simulink model "QRD_System"  (R2021a)
settings: Solver=VariableStepAuto  StartTime=0.0  StopTime=800  RelTol=1e-3
undefined symbols (not defined in the file or in its folder): AXI4, Lite
libraries: hdlBasic x268, xbsIndex_r4 x1
(part 2 of 3)

== system QRD_System/Rotation10 ==
  y_in : Inport
  theta_in : Inport  Port=2
  rst : Inport  Port=3
  Q_in : Inport  Port=4
  Constant3 : hdlBasic/Constant  const=0.0  gui_display_data_type=Fixed-point  arith_type=Signed (2's comp)  n_bits=16  bin_pt=13  preci_type=Single  exp_width=8  frac_width=24  explicit_period=off  period=1  XmcBlockStatus=1  maskContainerNames=tabcontainer1  block_type=constant  block_config=sysgen:Constant_config
  Constant4 : hdlBasic/Constant  const=1.0  gui_display_data_type=Boolean  arith_type=Boolean  n_bits=16  bin_pt=14  preci_type=Single  exp_width=8  frac_width=24  explicit_period=off  period=1  XmcBlockStatus=1  maskContainerNames=tabcontainer1  block_type=constant  block_config=sysgen:Constant_config
  Constant5 : hdlBasic/Constant  const=0  gui_display_data_type=Boolean  arith_type=Boolean  n_bits=16  bin_pt=14  preci_type=Single  exp_width=8  frac_width=24  explicit_period=off  period=1  XmcBlockStatus=1  maskContainerNames=tabcontainer1  block_type=constant  block_config=sysgen:Constant_config
  Constant6 : hdlBasic/Constant  const=0  gui_display_data_type=Boolean  arith_type=Boolean  n_bits=16  bin_pt=13  preci_type=Single  exp_width=8  frac_width=24  explicit_period=off  period=1  XmcBlockStatus=1  maskContainerNames=tabcontainer1  block_type=constant  block_config=sysgen:Constant_config
  Constant7 : hdlBasic/Constant  const=0.0  gui_display_data_type=Fixed-point  arith_type=Signed (2's comp)  n_bits=16  bin_pt=0  preci_type=Single  exp_width=8  frac_width=24  explicit_period=off  period=1  XmcBlockStatus=1  maskContainerNames=tabcontainer1  block_type=constant  block_config=sysgen:Constant_config
  Delay1 : hdlBasic/Delay  rst=off  en=off  latency=42  reg_retiming=off  XmcBlockStatus=1  maskContainerNames=group1  block_type=delay  block_config=sysgen:Delay_config
  Delay5 : hdlBasic/Delay  rst=off  en=off  latency=42  reg_retiming=off  XmcBlockStatus=1  maskContainerNames=group1  block_type=delay  block_config=sysgen:Delay_config
  Mux : hdlBasic/Mux  inputs=2  en=off  latency=0  precision=Full  arith_type=Unsigned  n_bits=16  bin_pt=14  quantization=Truncate  overflow=Wrap  XmcBlockStatus=1  maskContainerNames=tabcontainer1  block_type=mux  block_config=sysgen:Mux_config
  Mux2 : hdlBasic/Mux  inputs=2  en=off  latency=0  precision=Full  arith_type=Unsigned  n_bits=16  bin_pt=14  quantization=Truncate  overflow=Wrap  XmcBlockStatus=1  maskContainerNames=tabcontainer1  block_type=mux  block_config=sysgen:Mux_config
  Register : hdlBasic/Register  init=0  rst=on  en=off  XmcBlockStatus=1  maskContainerNames=tabcontainer1  block_type=register  block_config=sysgen:Register_config
  Scope6 : Scope
  Terminator{1..6} (6 alike) : Terminator
  Vitis HLS2 : hdlBasic/Vitis HLS  anytable='C:\ELEC522\hl116\Project5\project5_final\Vitis_HLS\project5_final_hls\solution1'  fast_sim=off  display_datatype=off  rate_propagation_method=Simulink system period  model_file_path=''  latency=1  block_type=vitis_hls
      settings: infoedit=This block allows including C,C++ and SystemC source files in System Generator for DSP designs.
  theta_out : Outport
  y_out : Outport  Port=2
  x_out : Outport  Port=3
  sel_out : Outport  Port=4
  Q_out : Outport  Port=5
  rst_out : Outport  Port=6
  wires:
  Mux/1 -> Mux2/3, Register/1
  Vitis HLS2/4 -> x_out/1, Mux/3
  y_in/1 -> Vitis HLS2/5
  Constant3/1 -> Mux/2
  Vitis HLS2/5 -> sel_out/1, Mux/1
  Vitis HLS2/6 -> y_out/1
  rst/1 -> Delay1/1, Register/2, Mux2/1
  Register/1 -> Vitis HLS2/4
  Constant6/1 -> Vitis HLS2/3
  Constant7/1 -> Vitis HLS2/7
  Constant4/1 -> Vitis HLS2/2
  Constant5/1 -> Vitis HLS2/1
  Vitis HLS2/1 -> Terminator3/1
  Vitis HLS2/2 -> Terminator1/1
  Vitis HLS2/3 -> Terminator6/1
  Vitis HLS2/7 -> Terminator2/1
  Vitis HLS2/8 -> Terminator5/1
  Vitis HLS2/9 -> Terminator4/1
  Mux2/1 -> Q_out/1, Scope6/1
  Q_in/1 -> Mux2/2
  Delay5/1 -> Vitis HLS2/6, theta_out/1
  theta_in/1 -> Delay5/1
  Delay1/1 -> rst_out/1

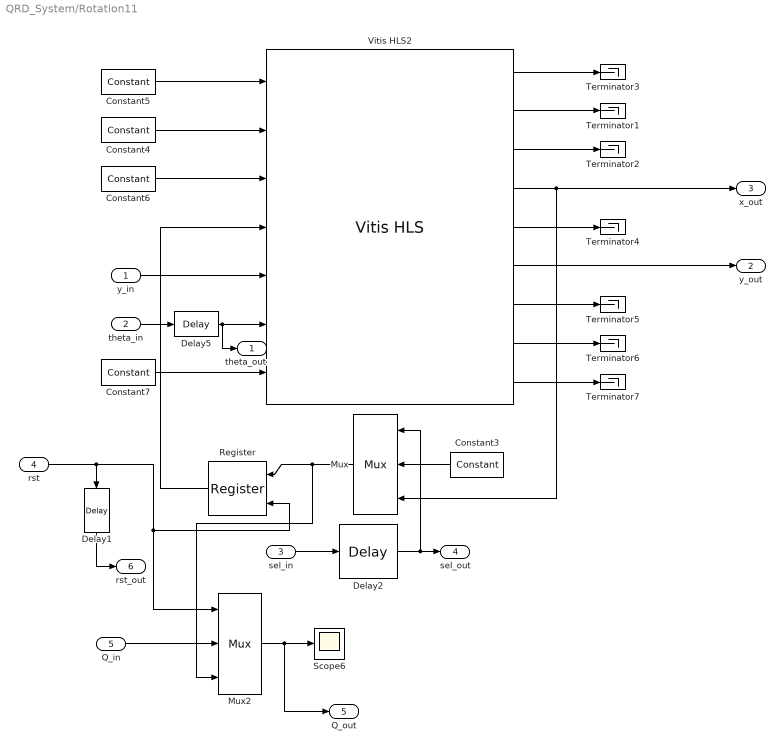
== system QRD_System/Rotation11 ==
  y_in : Inport
  theta_in : Inport  Port=2
  sel_in : Inport  Port=3
  rst : Inport  Port=4
  Q_in : Inport  Port=5
  Constant3 : hdlBasic/Constant  const=0.0  gui_display_data_type=Fixed-point  arith_type=Signed (2's comp)  n_bits=16  bin_pt=13  preci_type=Single  exp_width=8  frac_width=24  explicit_period=off  period=1  XmcBlockStatus=1  maskContainerNames=tabcontainer1  block_type=constant  block_config=sysgen:Constant_config
  Constant4 : hdlBasic/Constant  const=1.0  gui_display_data_type=Boolean  arith_type=Boolean  n_bits=16  bin_pt=14  preci_type=Single  exp_width=8  frac_width=24  explicit_period=off  period=1  XmcBlockStatus=1  maskContainerNames=tabcontainer1  block_type=constant  block_config=sysgen:Constant_config
  Constant5 : hdlBasic/Constant  const=0  gui_display_data_type=Boolean  arith_type=Boolean  n_bits=16  bin_pt=14  preci_type=Single  exp_width=8  frac_width=24  explicit_period=off  period=1  XmcBlockStatus=1  maskContainerNames=tabcontainer1  block_type=constant  block_config=sysgen:Constant_config
  Constant6 : hdlBasic/Constant  const=0  gui_display_data_type=Boolean  arith_type=Boolean  n_bits=16  bin_pt=13  preci_type=Single  exp_width=8  frac_width=24  explicit_period=off  period=1  XmcBlockStatus=1  maskContainerNames=tabcontainer1  block_type=constant  block_config=sysgen:Constant_config
  Constant7 : hdlBasic/Constant  const=0.0  gui_display_data_type=Fixed-point  arith_type=Signed (2's comp)  n_bits=16  bin_pt=0  preci_type=Single  exp_width=8  frac_width=24  explicit_period=off  period=1  XmcBlockStatus=1  maskContainerNames=tabcontainer1  block_type=constant  block_config=sysgen:Constant_config
  Delay1 : hdlBasic/Delay  rst=off  en=off  latency=42  reg_retiming=off  XmcBlockStatus=1  maskContainerNames=group1  block_type=delay  block_config=sysgen:Delay_config
  Delay2 : hdlBasic/Delay  rst=off  en=off  latency=43  reg_retiming=off  XmcBlockStatus=1  maskContainerNames=group1  block_type=delay  block_config=sysgen:Delay_config
  Delay5 : hdlBasic/Delay  rst=off  en=off  latency=42  reg_retiming=off  XmcBlockStatus=1  maskContainerNames=group1  block_type=delay  block_config=sysgen:Delay_config
  Mux : hdlBasic/Mux  inputs=2  en=off  latency=0  precision=Full  arith_type=Unsigned  n_bits=16  bin_pt=14  quantization=Truncate  overflow=Wrap  XmcBlockStatus=1  maskContainerNames=tabcontainer1  block_type=mux  block_config=sysgen:Mux_config
  Mux2 : hdlBasic/Mux  inputs=2  en=off  latency=0  precision=Full  arith_type=Unsigned  n_bits=16  bin_pt=14  quantization=Truncate  overflow=Wrap  XmcBlockStatus=1  maskContainerNames=tabcontainer1  block_type=mux  block_config=sysgen:Mux_config
  Register : hdlBasic/Register  init=0  rst=on  en=off  XmcBlockStatus=1  maskContainerNames=tabcontainer1  block_type=register  block_config=sysgen:Register_config
  Scope6 : Scope
  Terminator{1..7} (7 alike) : Terminator
  Vitis HLS2 : hdlBasic/Vitis HLS  anytable='C:\ELEC522\hl116\Project5\project5_final\Vitis_HLS\project5_final_hls\solution1'  fast_sim=off  display_datatype=off  rate_propagation_method=Simulink system period  model_file_path=''  latency=1  block_type=vitis_hls
      settings: infoedit=This block allows including C,C++ and SystemC source files in System Generator for DSP designs.
  theta_out : Outport
  y_out : Outport  Port=2
  x_out : Outport  Port=3
  sel_out : Outport  Port=4
  Q_out : Outport  Port=5
  rst_out : Outport  Port=6
  wires:
  Mux/1 -> Mux2/3, Register/1
  Vitis HLS2/4 -> x_out/1, Mux/3
  y_in/1 -> Vitis HLS2/5
  Constant3/1 -> Mux/2
  Vitis HLS2/6 -> y_out/1
  theta_in/1 -> Delay5/1
  sel_in/1 -> Delay2/1
  Register/1 -> Vitis HLS2/4
  rst/1 -> Delay1/1, Mux2/1, Register/2
  Delay2/1 -> Mux/1, sel_out/1
  Constant6/1 -> Vitis HLS2/3
  Constant7/1 -> Vitis HLS2/7
  Constant4/1 -> Vitis HLS2/2
  Constant5/1 -> Vitis HLS2/1
  Vitis HLS2/9 -> Terminator7/1
  Vitis HLS2/8 -> Terminator6/1
  Vitis HLS2/7 -> Terminator5/1
  Vitis HLS2/2 -> Terminator1/1
  Vitis HLS2/1 -> Terminator3/1
  Vitis HLS2/3 -> Terminator2/1
  Vitis HLS2/5 -> Terminator4/1
  Mux2/1 -> Q_out/1, Scope6/1
  Q_in/1 -> Mux2/2
  Delay5/1 -> Vitis HLS2/6, theta_out/1
  Delay1/1 -> rst_out/1

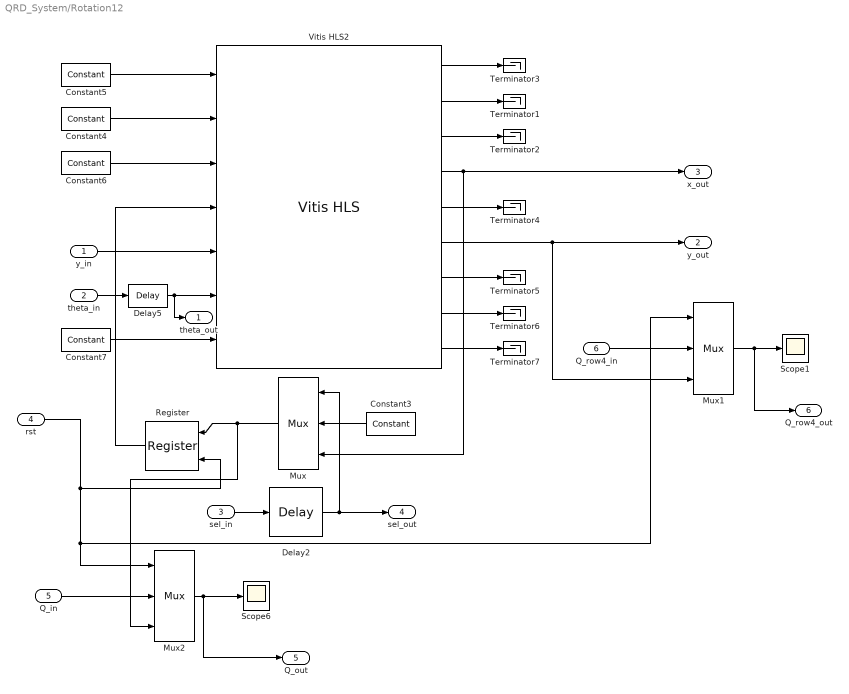
== system QRD_System/Rotation12 ==
  y_in : Inport
  theta_in : Inport  Port=2
  sel_in : Inport  Port=3
  rst : Inport  Port=4
  Q_in : Inport  Port=5
  Q_row4_in : Inport  Port=6
  Constant3 : hdlBasic/Constant  const=0.0  gui_display_data_type=Fixed-point  arith_type=Signed (2's comp)  n_bits=16  bin_pt=13  preci_type=Single  exp_width=8  frac_width=24  explicit_period=off  period=1  XmcBlockStatus=1  maskContainerNames=tabcontainer1  block_type=constant  block_config=sysgen:Constant_config
  Constant4 : hdlBasic/Constant  const=1.0  gui_display_data_type=Boolean  arith_type=Boolean  n_bits=16  bin_pt=14  preci_type=Single  exp_width=8  frac_width=24  explicit_period=off  period=1  XmcBlockStatus=1  maskContainerNames=tabcontainer1  block_type=constant  block_config=sysgen:Constant_config
  Constant5 : hdlBasic/Constant  const=0  gui_display_data_type=Boolean  arith_type=Boolean  n_bits=16  bin_pt=14  preci_type=Single  exp_width=8  frac_width=24  explicit_period=off  period=1  XmcBlockStatus=1  maskContainerNames=tabcontainer1  block_type=constant  block_config=sysgen:Constant_config
  Constant6 : hdlBasic/Constant  const=0  gui_display_data_type=Boolean  arith_type=Boolean  n_bits=16  bin_pt=13  preci_type=Single  exp_width=8  frac_width=24  explicit_period=off  period=1  XmcBlockStatus=1  maskContainerNames=tabcontainer1  block_type=constant  block_config=sysgen:Constant_config
  Constant7 : hdlBasic/Constant  const=0.0  gui_display_data_type=Fixed-point  arith_type=Signed (2's comp)  n_bits=16  bin_pt=0  preci_type=Single  exp_width=8  frac_width=24  explicit_period=off  period=1  XmcBlockStatus=1  maskContainerNames=tabcontainer1  block_type=constant  block_config=sysgen:Constant_config
  Delay2 : hdlBasic/Delay  rst=off  en=off  latency=43  reg_retiming=off  XmcBlockStatus=1  maskContainerNames=group1  block_type=delay  block_config=sysgen:Delay_config
  Delay5 : hdlBasic/Delay  rst=off  en=off  latency=42  reg_retiming=off  XmcBlockStatus=1  maskContainerNames=group1  block_type=delay  block_config=sysgen:Delay_config
  Mux : hdlBasic/Mux  inputs=2  en=off  latency=0  precision=Full  arith_type=Unsigned  n_bits=16  bin_pt=14  quantization=Truncate  overflow=Wrap  XmcBlockStatus=1  maskContainerNames=tabcontainer1  block_type=mux  block_config=sysgen:Mux_config
  Mux1 : hdlBasic/Mux  inputs=2  en=off  latency=0  precision=Full  arith_type=Unsigned  n_bits=16  bin_pt=14  quantization=Truncate  overflow=Wrap  XmcBlockStatus=1  maskContainerNames=tabcontainer1  block_type=mux  block_config=sysgen:Mux_config
  Mux2 : hdlBasic/Mux  inputs=2  en=off  latency=0  precision=Full  arith_type=Unsigned  n_bits=16  bin_pt=14  quantization=Truncate  overflow=Wrap  XmcBlockStatus=1  maskContainerNames=tabcontainer1  block_type=mux  block_config=sysgen:Mux_config
  Register : hdlBasic/Register  init=0  rst=on  en=off  XmcBlockStatus=1  maskContainerNames=tabcontainer1  block_type=register  block_config=sysgen:Register_config
  Scope1 : Scope
  Scope6 : Scope
  Terminator{1..7} (7 alike) : Terminator
  Vitis HLS2 : hdlBasic/Vitis HLS  anytable='C:\ELEC522\hl116\Project5\project5_final\Vitis_HLS\project5_final_hls\solution1'  fast_sim=off  display_datatype=off  rate_propagation_method=Simulink system period  model_file_path=''  latency=1  block_type=vitis_hls
      settings: infoedit=This block allows including C,C++ and SystemC source files in System Generator for DSP designs.
  theta_out : Outport
  y_out : Outport  Port=2
  x_out : Outport  Port=3
  sel_out : Outport  Port=4
  Q_out : Outport  Port=5
  Q_row4_out : Outport  Port=6
  wires:
  Mux/1 -> Mux2/3, Register/1
  Vitis HLS2/4 -> x_out/1, Mux/3
  y_in/1 -> Vitis HLS2/5
  Constant3/1 -> Mux/2
  theta_in/1 -> Delay5/1
  sel_in/1 -> Delay2/1
  Register/1 -> Vitis HLS2/4
  rst/1 -> Mux2/1, Mux1/1, Register/2
  Delay2/1 -> Mux/1, sel_out/1
  Constant6/1 -> Vitis HLS2/3
  Constant7/1 -> Vitis HLS2/7
  Constant4/1 -> Vitis HLS2/2
  Constant5/1 -> Vitis HLS2/1
  Vitis HLS2/3 -> Terminator2/1
  Vitis HLS2/2 -> Terminator1/1
  Vitis HLS2/1 -> Terminator3/1
  Vitis HLS2/5 -> Terminator4/1
  Vitis HLS2/7 -> Terminator5/1
  Vitis HLS2/8 -> Terminator6/1
  Vitis HLS2/9 -> Terminator7/1
  Mux1/1 -> Q_row4_out/1, Scope1/1
  Q_row4_in/1 -> Mux1/2
  Vitis HLS2/6 -> Mux1/3, y_out/1
  Q_in/1 -> Mux2/2
  Mux2/1 -> Q_out/1, Scope6/1
  Delay5/1 -> Vitis HLS2/6, theta_out/1

== system QRD_System/Rotation13 ==
  y_in : Inport
  theta_in : Inport  Port=2
  rst : Inport  Port=3
  Q_in : Inport  Port=4
  Constant3 : hdlBasic/Constant  const=0.0  gui_display_data_type=Fixed-point  arith_type=Signed (2's comp)  n_bits=16  bin_pt=13  preci_type=Single  exp_width=8  frac_width=24  explicit_period=off  period=1  XmcBlockStatus=1  maskContainerNames=tabcontainer1  block_type=constant  block_config=sysgen:Constant_config
  Constant4 : hdlBasic/Constant  const=1.0  gui_display_data_type=Boolean  arith_type=Boolean  n_bits=16  bin_pt=14  preci_type=Single  exp_width=8  frac_width=24  explicit_period=off  period=1  XmcBlockStatus=1  maskContainerNames=tabcontainer1  block_type=constant  block_config=sysgen:Constant_config
  Constant5 : hdlBasic/Constant  const=0  gui_display_data_type=Boolean  arith_type=Boolean  n_bits=16  bin_pt=14  preci_type=Single  exp_width=8  frac_width=24  explicit_period=off  period=1  XmcBlockStatus=1  maskContainerNames=tabcontainer1  block_type=constant  block_config=sysgen:Constant_config
  Constant6 : hdlBasic/Constant  const=0  gui_display_data_type=Boolean  arith_type=Boolean  n_bits=16  bin_pt=13  preci_type=Single  exp_width=8  frac_width=24  explicit_period=off  period=1  XmcBlockStatus=1  maskContainerNames=tabcontainer1  block_type=constant  block_config=sysgen:Constant_config
  Constant7 : hdlBasic/Constant  const=0.0  gui_display_data_type=Fixed-point  arith_type=Signed (2's comp)  n_bits=16  bin_pt=0  preci_type=Single  exp_width=8  frac_width=24  explicit_period=off  period=1  XmcBlockStatus=1  maskContainerNames=tabcontainer1  block_type=constant  block_config=sysgen:Constant_config
  Delay1 : hdlBasic/Delay  rst=off  en=off  latency=42  reg_retiming=off  XmcBlockStatus=1  maskContainerNames=group1  block_type=delay  block_config=sysgen:Delay_config
  Delay5 : hdlBasic/Delay  rst=off  en=off  latency=42  reg_retiming=off  XmcBlockStatus=1  maskContainerNames=group1  block_type=delay  block_config=sysgen:Delay_config
  Mux : hdlBasic/Mux  inputs=2  en=off  latency=0  precision=Full  arith_type=Unsigned  n_bits=16  bin_pt=14  quantization=Truncate  overflow=Wrap  XmcBlockStatus=1  maskContainerNames=tabcontainer1  block_type=mux  block_config=sysgen:Mux_config
  Mux2 : hdlBasic/Mux  inputs=2  en=off  latency=0  precision=Full  arith_type=Unsigned  n_bits=16  bin_pt=14  quantization=Truncate  overflow=Wrap  XmcBlockStatus=1  maskContainerNames=tabcontainer1  block_type=mux  block_config=sysgen:Mux_config
  Register : hdlBasic/Register  init=0  rst=on  en=off  XmcBlockStatus=1  maskContainerNames=tabcontainer1  block_type=register  block_config=sysgen:Register_config
  Scope6 : Scope
  Terminator{1..6} (6 alike) : Terminator
  Vitis HLS2 : hdlBasic/Vitis HLS  anytable='C:\ELEC522\hl116\Project5\project5_final\Vitis_HLS\project5_final_hls\solution1'  fast_sim=off  display_datatype=off  rate_propagation_method=Simulink system period  model_file_path=''  latency=1  block_type=vitis_hls
      settings: infoedit=This block allows including C,C++ and SystemC source files in System Generator for DSP designs.
  theta_out : Outport
  y_out : Outport  Port=2
  x_out : Outport  Port=3
  sel_out : Outport  Port=4
  Q_out : Outport  Port=5
  rst_out : Outport  Port=6
  wires:
  Mux/1 -> Mux2/3, Register/1
  Vitis HLS2/4 -> Mux/3, x_out/1
  y_in/1 -> Vitis HLS2/5
  Constant3/1 -> Mux/2
  Vitis HLS2/5 -> sel_out/1, Mux/1
  Vitis HLS2/6 -> y_out/1
  rst/1 -> Delay1/1, Register/2, Mux2/1
  Register/1 -> Vitis HLS2/4
  Constant6/1 -> Vitis HLS2/3
  Constant7/1 -> Vitis HLS2/7
  Constant4/1 -> Vitis HLS2/2
  Constant5/1 -> Vitis HLS2/1
  Vitis HLS2/7 -> Terminator2/1
  Vitis HLS2/8 -> Terminator5/1
  Vitis HLS2/9 -> Terminator4/1
  Vitis HLS2/3 -> Terminator6/1
  Vitis HLS2/2 -> Terminator1/1
  Vitis HLS2/1 -> Terminator3/1
  Mux2/1 -> Q_out/1, Scope6/1
  Q_in/1 -> Mux2/2
  Delay5/1 -> Vitis HLS2/6, theta_out/1
  theta_in/1 -> Delay5/1
  Delay1/1 -> rst_out/1

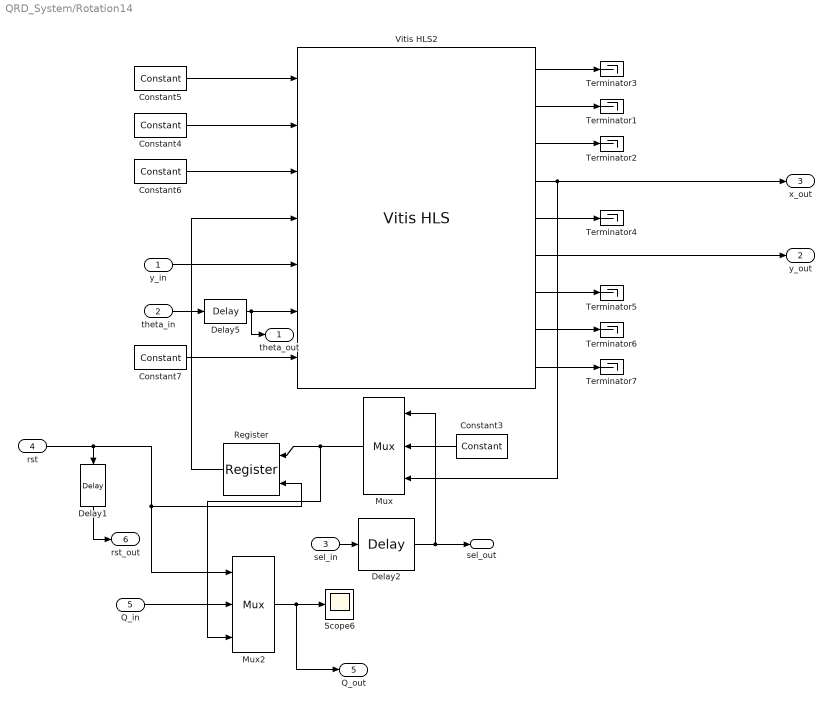
== system QRD_System/Rotation14 ==
  y_in : Inport
  theta_in : Inport  Port=2
  sel_in : Inport  Port=3
  rst : Inport  Port=4
  Q_in : Inport  Port=5
  Constant3 : hdlBasic/Constant  const=0.0  gui_display_data_type=Fixed-point  arith_type=Signed (2's comp)  n_bits=16  bin_pt=13  preci_type=Single  exp_width=8  frac_width=24  explicit_period=off  period=1  XmcBlockStatus=1  maskContainerNames=tabcontainer1  block_type=constant  block_config=sysgen:Constant_config
  Constant4 : hdlBasic/Constant  const=1.0  gui_display_data_type=Boolean  arith_type=Boolean  n_bits=16  bin_pt=14  preci_type=Single  exp_width=8  frac_width=24  explicit_period=off  period=1  XmcBlockStatus=1  maskContainerNames=tabcontainer1  block_type=constant  block_config=sysgen:Constant_config
  Constant5 : hdlBasic/Constant  const=0  gui_display_data_type=Boolean  arith_type=Boolean  n_bits=16  bin_pt=14  preci_type=Single  exp_width=8  frac_width=24  explicit_period=off  period=1  XmcBlockStatus=1  maskContainerNames=tabcontainer1  block_type=constant  block_config=sysgen:Constant_config
  Constant6 : hdlBasic/Constant  const=0  gui_display_data_type=Boolean  arith_type=Boolean  n_bits=16  bin_pt=13  preci_type=Single  exp_width=8  frac_width=24  explicit_period=off  period=1  XmcBlockStatus=1  maskContainerNames=tabcontainer1  block_type=constant  block_config=sysgen:Constant_config
  Constant7 : hdlBasic/Constant  const=0.0  gui_display_data_type=Fixed-point  arith_type=Signed (2's comp)  n_bits=16  bin_pt=0  preci_type=Single  exp_width=8  frac_width=24  explicit_period=off  period=1  XmcBlockStatus=1  maskContainerNames=tabcontainer1  block_type=constant  block_config=sysgen:Constant_config
  Delay1 : hdlBasic/Delay  rst=off  en=off  latency=42  reg_retiming=off  XmcBlockStatus=1  maskContainerNames=group1  block_type=delay  block_config=sysgen:Delay_config
  Delay2 : hdlBasic/Delay  rst=off  en=off  latency=43  reg_retiming=off  XmcBlockStatus=1  maskContainerNames=group1  block_type=delay  block_config=sysgen:Delay_config
  Delay5 : hdlBasic/Delay  rst=off  en=off  latency=42  reg_retiming=off  XmcBlockStatus=1  maskContainerNames=group1  block_type=delay  block_config=sysgen:Delay_config
  Mux : hdlBasic/Mux  inputs=2  en=off  latency=0  precision=Full  arith_type=Unsigned  n_bits=16  bin_pt=14  quantization=Truncate  overflow=Wrap  XmcBlockStatus=1  maskContainerNames=tabcontainer1  block_type=mux  block_config=sysgen:Mux_config
  Mux2 : hdlBasic/Mux  inputs=2  en=off  latency=0  precision=Full  arith_type=Unsigned  n_bits=16  bin_pt=14  quantization=Truncate  overflow=Wrap  XmcBlockStatus=1  maskContainerNames=tabcontainer1  block_type=mux  block_config=sysgen:Mux_config
  Register : hdlBasic/Register  init=0  rst=on  en=off  XmcBlockStatus=1  maskContainerNames=tabcontainer1  block_type=register  block_config=sysgen:Register_config
  Scope6 : Scope
  Terminator{1..7} (7 alike) : Terminator
  Vitis HLS2 : hdlBasic/Vitis HLS  anytable='C:\ELEC522\hl116\Project5\project5_final\Vitis_HLS\project5_final_hls\solution1'  fast_sim=off  display_datatype=off  rate_propagation_method=Simulink system period  model_file_path=''  latency=1  block_type=vitis_hls
      settings: infoedit=This block allows including C,C++ and SystemC source files in System Generator for DSP designs.
  theta_out : Outport
  y_out : Outport  Port=2
  x_out : Outport  Port=3
  sel_out : Outport  Port=4
  Q_out : Outport  Port=5
  rst_out : Outport  Port=6
  wires:
  Mux/1 -> Mux2/3, Register/1
  Vitis HLS2/4 -> Mux/3, x_out/1
  Constant3/1 -> Mux/2
  Vitis HLS2/6 -> y_out/1
  theta_in/1 -> Delay5/1
  Register/1 -> Vitis HLS2/4
  rst/1 -> Delay1/1, Mux2/1, Register/2
  Constant6/1 -> Vitis HLS2/3
  Constant7/1 -> Vitis HLS2/7
  Constant4/1 -> Vitis HLS2/2
  Constant5/1 -> Vitis HLS2/1
  y_in/1 -> Vitis HLS2/5
  Vitis HLS2/7 -> Terminator5/1
  Vitis HLS2/8 -> Terminator6/1
  Vitis HLS2/1 -> Terminator3/1
  Vitis HLS2/2 -> Terminator1/1
  Vitis HLS2/3 -> Terminator2/1
  Vitis HLS2/5 -> Terminator4/1
  Vitis HLS2/9 -> Terminator7/1
  sel_in/1 -> Delay2/1
  Delay2/1 -> sel_out/1, Mux/1
  Mux2/1 -> Q_out/1, Scope6/1
  Q_in/1 -> Mux2/2
  Delay5/1 -> theta_out/1, Vitis HLS2/6
  Delay1/1 -> rst_out/1

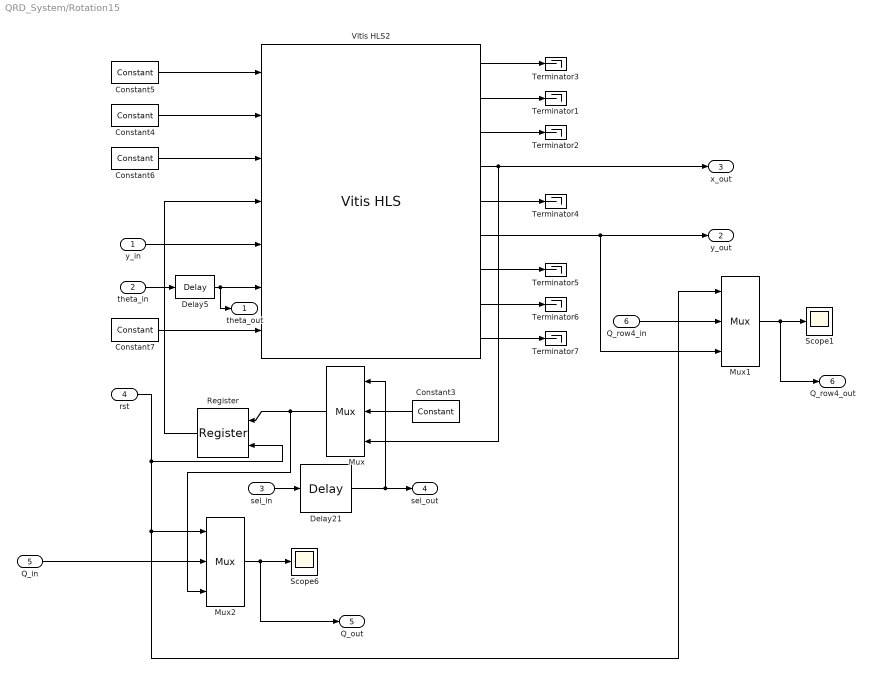
== system QRD_System/Rotation15 ==
  y_in : Inport
  theta_in : Inport  Port=2
  sel_in : Inport  Port=3
  rst : Inport  Port=4
  Q_in : Inport  Port=5
  Q_row4_in : Inport  Port=6
  Constant3 : hdlBasic/Constant  const=0.0  gui_display_data_type=Fixed-point  arith_type=Signed (2's comp)  n_bits=16  bin_pt=13  preci_type=Single  exp_width=8  frac_width=24  explicit_period=off  period=1  XmcBlockStatus=1  maskContainerNames=tabcontainer1  block_type=constant  block_config=sysgen:Constant_config
  Constant4 : hdlBasic/Constant  const=1.0  gui_display_data_type=Boolean  arith_type=Boolean  n_bits=16  bin_pt=14  preci_type=Single  exp_width=8  frac_width=24  explicit_period=off  period=1  XmcBlockStatus=1  maskContainerNames=tabcontainer1  block_type=constant  block_config=sysgen:Constant_config
  Constant5 : hdlBasic/Constant  const=0  gui_display_data_type=Boolean  arith_type=Boolean  n_bits=16  bin_pt=14  preci_type=Single  exp_width=8  frac_width=24  explicit_period=off  period=1  XmcBlockStatus=1  maskContainerNames=tabcontainer1  block_type=constant  block_config=sysgen:Constant_config
  Constant6 : hdlBasic/Constant  const=0  gui_display_data_type=Boolean  arith_type=Boolean  n_bits=16  bin_pt=13  preci_type=Single  exp_width=8  frac_width=24  explicit_period=off  period=1  XmcBlockStatus=1  maskContainerNames=tabcontainer1  block_type=constant  block_config=sysgen:Constant_config
  Constant7 : hdlBasic/Constant  const=0.0  gui_display_data_type=Fixed-point  arith_type=Signed (2's comp)  n_bits=16  bin_pt=0  preci_type=Single  exp_width=8  frac_width=24  explicit_period=off  period=1  XmcBlockStatus=1  maskContainerNames=tabcontainer1  block_type=constant  block_config=sysgen:Constant_config
  Delay21 : hdlBasic/Delay  rst=off  en=off  latency=43  reg_retiming=off  XmcBlockStatus=1  maskContainerNames=group1  block_type=delay  block_config=sysgen:Delay_config
  Delay5 : hdlBasic/Delay  rst=off  en=off  latency=42  reg_retiming=off  XmcBlockStatus=1  maskContainerNames=group1  block_type=delay  block_config=sysgen:Delay_config
  Mux : hdlBasic/Mux  inputs=2  en=off  latency=0  precision=Full  arith_type=Unsigned  n_bits=16  bin_pt=14  quantization=Truncate  overflow=Wrap  XmcBlockStatus=1  maskContainerNames=tabcontainer1  block_type=mux  block_config=sysgen:Mux_config
  Mux1 : hdlBasic/Mux  inputs=2  en=off  latency=0  precision=Full  arith_type=Unsigned  n_bits=16  bin_pt=14  quantization=Truncate  overflow=Wrap  XmcBlockStatus=1  maskContainerNames=tabcontainer1  block_type=mux  block_config=sysgen:Mux_config
  Mux2 : hdlBasic/Mux  inputs=2  en=off  latency=0  precision=Full  arith_type=Unsigned  n_bits=16  bin_pt=14  quantization=Truncate  overflow=Wrap  XmcBlockStatus=1  maskContainerNames=tabcontainer1  block_type=mux  block_config=sysgen:Mux_config
  Register : hdlBasic/Register  init=0  rst=on  en=off  XmcBlockStatus=1  maskContainerNames=tabcontainer1  block_type=register  block_config=sysgen:Register_config
  Scope1 : Scope
  Scope6 : Scope
  Terminator{1..7} (7 alike) : Terminator
  Vitis HLS2 : hdlBasic/Vitis HLS  anytable='C:\ELEC522\hl116\Project5\project5_final\Vitis_HLS\project5_final_hls\solution1'  fast_sim=off  display_datatype=off  rate_propagation_method=Simulink system period  model_file_path=''  latency=1  block_type=vitis_hls
      settings: infoedit=This block allows including C,C++ and SystemC source files in System Generator for DSP designs.
  theta_out : Outport
  y_out : Outport  Port=2
  x_out : Outport  Port=3
  sel_out : Outport  Port=4
  Q_out : Outport  Port=5
  Q_row4_out : Outport  Port=6
  wires:
  Mux/1 -> Mux2/3, Register/1
  Vitis HLS2/4 -> x_out/1, Mux/3
  y_in/1 -> Vitis HLS2/5
  Constant3/1 -> Mux/2
  theta_in/1 -> Delay5/1
  sel_in/1 -> Delay21/1
  Register/1 -> Vitis HLS2/4
  Delay21/1 -> Mux/1, sel_out/1
  Constant6/1 -> Vitis HLS2/3
  Constant7/1 -> Vitis HLS2/7
  Constant4/1 -> Vitis HLS2/2
  Constant5/1 -> Vitis HLS2/1
  Vitis HLS2/1 -> Terminator3/1
  Vitis HLS2/2 -> Terminator1/1
  Vitis HLS2/3 -> Terminator2/1
  Vitis HLS2/5 -> Terminator4/1
  Vitis HLS2/7 -> Terminator5/1
  Vitis HLS2/8 -> Terminator6/1
  Vitis HLS2/9 -> Terminator7/1
  Q_in/1 -> Mux2/2
  rst/1 -> Mux1/1, Mux2/1, Register/2
  Mux1/1 -> Q_row4_out/1, Scope1/1
  Q_row4_in/1 -> Mux1/2
  Vitis HLS2/6 -> Mux1/3, y_out/1
  Mux2/1 -> Q_out/1, Scope6/1
  Delay5/1 -> theta_out/1, Vitis HLS2/6

== system QRD_System/Rotation16 ==
  y_in : Inport
  theta_in : Inport  Port=2
  rst : Inport  Port=3
  Q_in : Inport  Port=4
  Constant3 : hdlBasic/Constant  const=0.0  gui_display_data_type=Fixed-point  arith_type=Signed (2's comp)  n_bits=16  bin_pt=13  preci_type=Single  exp_width=8  frac_width=24  explicit_period=off  period=1  XmcBlockStatus=1  maskContainerNames=tabcontainer1  block_type=constant  block_config=sysgen:Constant_config
  Constant4 : hdlBasic/Constant  const=1.0  gui_display_data_type=Boolean  arith_type=Boolean  n_bits=16  bin_pt=14  preci_type=Single  exp_width=8  frac_width=24  explicit_period=off  period=1  XmcBlockStatus=1  maskContainerNames=tabcontainer1  block_type=constant  block_config=sysgen:Constant_config
  Constant5 : hdlBasic/Constant  const=0  gui_display_data_type=Boolean  arith_type=Boolean  n_bits=16  bin_pt=14  preci_type=Single  exp_width=8  frac_width=24  explicit_period=off  period=1  XmcBlockStatus=1  maskContainerNames=tabcontainer1  block_type=constant  block_config=sysgen:Constant_config
  Constant6 : hdlBasic/Constant  const=0  gui_display_data_type=Boolean  arith_type=Boolean  n_bits=16  bin_pt=13  preci_type=Single  exp_width=8  frac_width=24  explicit_period=off  period=1  XmcBlockStatus=1  maskContainerNames=tabcontainer1  block_type=constant  block_config=sysgen:Constant_config
  Constant7 : hdlBasic/Constant  const=0.0  gui_display_data_type=Fixed-point  arith_type=Signed (2's comp)  n_bits=16  bin_pt=0  preci_type=Single  exp_width=8  frac_width=24  explicit_period=off  period=1  XmcBlockStatus=1  maskContainerNames=tabcontainer1  block_type=constant  block_config=sysgen:Constant_config
  Delay1 : hdlBasic/Delay  rst=off  en=off  latency=42  reg_retiming=off  XmcBlockStatus=1  maskContainerNames=group1  block_type=delay  block_config=sysgen:Delay_config
  Delay5 : hdlBasic/Delay  rst=off  en=off  latency=42  reg_retiming=off  XmcBlockStatus=1  maskContainerNames=group1  block_type=delay  block_config=sysgen:Delay_config
  Mux : hdlBasic/Mux  inputs=2  en=off  latency=0  precision=Full  arith_type=Unsigned  n_bits=16  bin_pt=14  quantization=Truncate  overflow=Wrap  XmcBlockStatus=1  maskContainerNames=tabcontainer1  block_type=mux  block_config=sysgen:Mux_config
  Mux2 : hdlBasic/Mux  inputs=2  en=off  latency=0  precision=Full  arith_type=Unsigned  n_bits=16  bin_pt=14  quantization=Truncate  overflow=Wrap  XmcBlockStatus=1  maskContainerNames=tabcontainer1  block_type=mux  block_config=sysgen:Mux_config
  Register : hdlBasic/Register  init=0  rst=on  en=off  XmcBlockStatus=1  maskContainerNames=tabcontainer1  block_type=register  block_config=sysgen:Register_config
  Scope6 : Scope
  Terminator{1..6} (6 alike) : Terminator
  Vitis HLS2 : hdlBasic/Vitis HLS  anytable='C:\ELEC522\hl116\Project5\project5_final\Vitis_HLS\project5_final_hls\solution1'  fast_sim=off  display_datatype=off  rate_propagation_method=Simulink system period  model_file_path=''  latency=1  block_type=vitis_hls
      settings: infoedit=This block allows including C,C++ and SystemC source files in System Generator for DSP designs.
  theta_out : Outport
  y_out : Outport  Port=2
  x_out : Outport  Port=3
  sel_out : Outport  Port=4
  Q_out : Outport  Port=5
  rst_out : Outport  Port=6
  wires:
  Mux/1 -> Mux2/3, Register/1
  Vitis HLS2/4 -> Mux/3, x_out/1
  y_in/1 -> Vitis HLS2/5
  Constant3/1 -> Mux/2
  Vitis HLS2/5 -> Mux/1, sel_out/1
  Vitis HLS2/6 -> y_out/1
  rst/1 -> Delay1/1, Register/2, Mux2/1
  Register/1 -> Vitis HLS2/4
  Constant6/1 -> Vitis HLS2/3
  Constant7/1 -> Vitis HLS2/7
  Constant4/1 -> Vitis HLS2/2
  Constant5/1 -> Vitis HLS2/1
  Vitis HLS2/1 -> Terminator3/1
  Vitis HLS2/2 -> Terminator1/1
  Vitis HLS2/3 -> Terminator6/1
  Vitis HLS2/7 -> Terminator2/1
  Vitis HLS2/8 -> Terminator5/1
  Vitis HLS2/9 -> Terminator4/1
  Mux2/1 -> Q_out/1, Scope6/1
  Q_in/1 -> Mux2/2
  Delay5/1 -> Vitis HLS2/6, theta_out/1
  theta_in/1 -> Delay5/1
  Delay1/1 -> rst_out/1

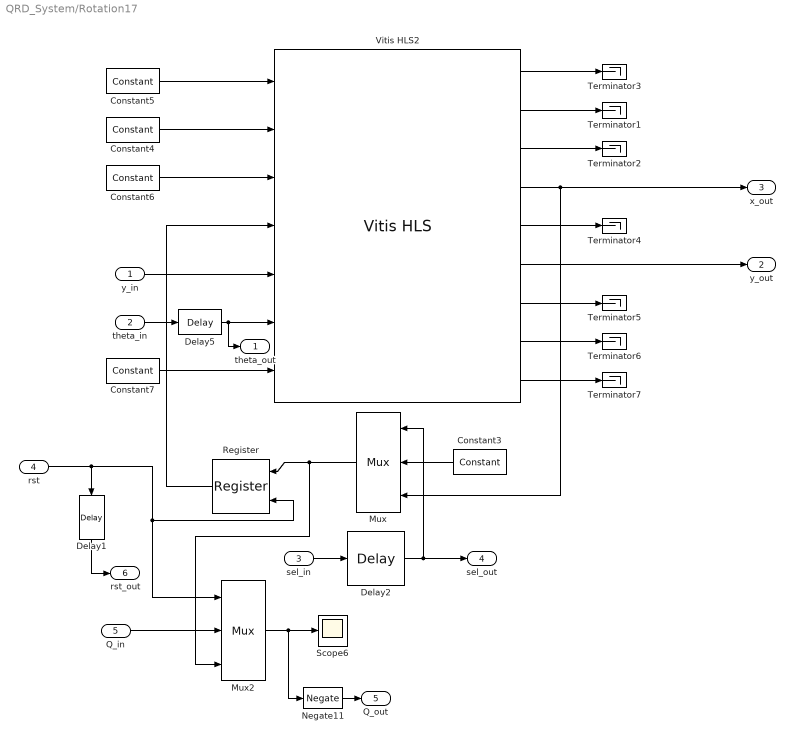
== system QRD_System/Rotation17 ==
  y_in : Inport
  theta_in : Inport  Port=2
  sel_in : Inport  Port=3
  rst : Inport  Port=4
  Q_in : Inport  Port=5
  Constant3 : hdlBasic/Constant  const=0.0  gui_display_data_type=Fixed-point  arith_type=Signed (2's comp)  n_bits=16  bin_pt=13  preci_type=Single  exp_width=8  frac_width=24  explicit_period=off  period=1  XmcBlockStatus=1  maskContainerNames=tabcontainer1  block_type=constant  block_config=sysgen:Constant_config
  Constant4 : hdlBasic/Constant  const=1.0  gui_display_data_type=Boolean  arith_type=Boolean  n_bits=16  bin_pt=14  preci_type=Single  exp_width=8  frac_width=24  explicit_period=off  period=1  XmcBlockStatus=1  maskContainerNames=tabcontainer1  block_type=constant  block_config=sysgen:Constant_config
  Constant5 : hdlBasic/Constant  const=0  gui_display_data_type=Boolean  arith_type=Boolean  n_bits=16  bin_pt=14  preci_type=Single  exp_width=8  frac_width=24  explicit_period=off  period=1  XmcBlockStatus=1  maskContainerNames=tabcontainer1  block_type=constant  block_config=sysgen:Constant_config
  Constant6 : hdlBasic/Constant  const=0  gui_display_data_type=Boolean  arith_type=Boolean  n_bits=16  bin_pt=13  preci_type=Single  exp_width=8  frac_width=24  explicit_period=off  period=1  XmcBlockStatus=1  maskContainerNames=tabcontainer1  block_type=constant  block_config=sysgen:Constant_config
  Constant7 : hdlBasic/Constant  const=0.0  gui_display_data_type=Fixed-point  arith_type=Signed (2's comp)  n_bits=16  bin_pt=0  preci_type=Single  exp_width=8  frac_width=24  explicit_period=off  period=1  XmcBlockStatus=1  maskContainerNames=tabcontainer1  block_type=constant  block_config=sysgen:Constant_config
  Delay1 : hdlBasic/Delay  rst=off  en=off  latency=42  reg_retiming=off  XmcBlockStatus=1  maskContainerNames=group1  block_type=delay  block_config=sysgen:Delay_config
  Delay2 : hdlBasic/Delay  rst=off  en=off  latency=43  reg_retiming=off  XmcBlockStatus=1  maskContainerNames=group1  block_type=delay  block_config=sysgen:Delay_config
  Delay5 : hdlBasic/Delay  rst=off  en=off  latency=42  reg_retiming=off  XmcBlockStatus=1  maskContainerNames=group1  block_type=delay  block_config=sysgen:Delay_config
  Mux : hdlBasic/Mux  inputs=2  en=off  latency=0  precision=Full  arith_type=Unsigned  n_bits=16  bin_pt=14  quantization=Truncate  overflow=Wrap  XmcBlockStatus=1  maskContainerNames=tabcontainer1  block_type=mux  block_config=sysgen:Mux_config
  Mux2 : hdlBasic/Mux  inputs=2  en=off  latency=0  precision=Full  arith_type=Unsigned  n_bits=16  bin_pt=14  quantization=Truncate  overflow=Wrap  XmcBlockStatus=1  maskContainerNames=tabcontainer1  block_type=mux  block_config=sysgen:Mux_config
  Negate11 : hdlBasic/Negate  precision=User Defined  arith_type="Signed  (2's comp)"  n_bits=16  bin_pt=13  quantization=Truncate  overflow=Wrap  en=off  latency=0  XmcBlockStatus=1  maskContainerNames=tabcontainer1  block_type=negate  block_config=sysgen:Negate_config
  Register : hdlBasic/Register  init=0  rst=on  en=off  XmcBlockStatus=1  maskContainerNames=tabcontainer1  block_type=register  block_config=sysgen:Register_config
  Scope6 : Scope
  Terminator{1..7} (7 alike) : Terminator
  Vitis HLS2 : hdlBasic/Vitis HLS  anytable='C:\ELEC522\hl116\Project5\project5_final\Vitis_HLS\project5_final_hls\solution1'  fast_sim=off  display_datatype=off  rate_propagation_method=Simulink system period  model_file_path=''  latency=1  block_type=vitis_hls
      settings: infoedit=This block allows including C,C++ and SystemC source files in System Generator for DSP designs.
  theta_out : Outport
  y_out : Outport  Port=2
  x_out : Outport  Port=3
  sel_out : Outport  Port=4
  Q_out : Outport  Port=5
  rst_out : Outport  Port=6
  wires:
  Mux/1 -> Mux2/3, Register/1
  Vitis HLS2/4 -> x_out/1, Mux/3
  y_in/1 -> Vitis HLS2/5
  Constant3/1 -> Mux/2
  Vitis HLS2/6 -> y_out/1
  theta_in/1 -> Delay5/1
  sel_in/1 -> Delay2/1
  Register/1 -> Vitis HLS2/4
  rst/1 -> Delay1/1, Mux2/1, Register/2
  Delay2/1 -> Mux/1, sel_out/1
  Constant6/1 -> Vitis HLS2/3
  Constant7/1 -> Vitis HLS2/7
  Constant4/1 -> Vitis HLS2/2
  Constant5/1 -> Vitis HLS2/1
  Vitis HLS2/1 -> Terminator3/1
  Vitis HLS2/2 -> Terminator1/1
  Vitis HLS2/3 -> Terminator2/1
  Vitis HLS2/5 -> Terminator4/1
  Vitis HLS2/7 -> Terminator5/1
  Vitis HLS2/8 -> Terminator6/1
  Vitis HLS2/9 -> Terminator7/1
  Mux2/1 -> Negate11/1, Scope6/1
  Q_in/1 -> Mux2/2
  Delay5/1 -> theta_out/1, Vitis HLS2/6
  Delay1/1 -> rst_out/1
  Negate11/1 -> Q_out/1

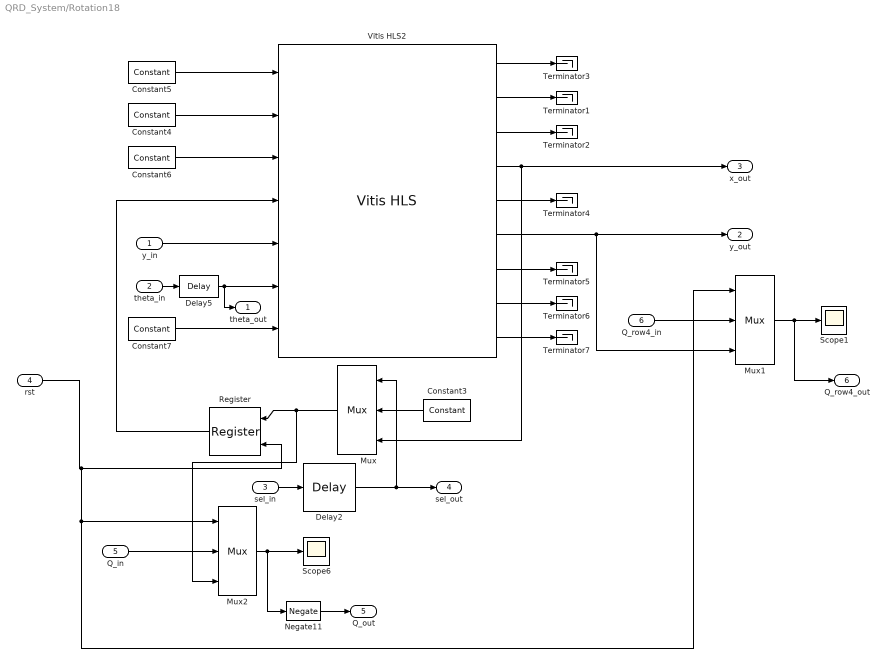
== system QRD_System/Rotation18 ==
  y_in : Inport
  theta_in : Inport  Port=2
  sel_in : Inport  Port=3
  rst : Inport  Port=4
  Q_in : Inport  Port=5
  Q_row4_in : Inport  Port=6
  Constant3 : hdlBasic/Constant  const=0.0  gui_display_data_type=Fixed-point  arith_type=Signed (2's comp)  n_bits=16  bin_pt=13  preci_type=Single  exp_width=8  frac_width=24  explicit_period=off  period=1  XmcBlockStatus=1  maskContainerNames=tabcontainer1  block_type=constant  block_config=sysgen:Constant_config
  Constant4 : hdlBasic/Constant  const=1.0  gui_display_data_type=Boolean  arith_type=Boolean  n_bits=16  bin_pt=14  preci_type=Single  exp_width=8  frac_width=24  explicit_period=off  period=1  XmcBlockStatus=1  maskContainerNames=tabcontainer1  block_type=constant  block_config=sysgen:Constant_config
  Constant5 : hdlBasic/Constant  const=0  gui_display_data_type=Boolean  arith_type=Boolean  n_bits=16  bin_pt=14  preci_type=Single  exp_width=8  frac_width=24  explicit_period=off  period=1  XmcBlockStatus=1  maskContainerNames=tabcontainer1  block_type=constant  block_config=sysgen:Constant_config
  Constant6 : hdlBasic/Constant  const=0  gui_display_data_type=Boolean  arith_type=Boolean  n_bits=16  bin_pt=13  preci_type=Single  exp_width=8  frac_width=24  explicit_period=off  period=1  XmcBlockStatus=1  maskContainerNames=tabcontainer1  block_type=constant  block_config=sysgen:Constant_config
  Constant7 : hdlBasic/Constant  const=0.0  gui_display_data_type=Fixed-point  arith_type=Signed (2's comp)  n_bits=16  bin_pt=0  preci_type=Single  exp_width=8  frac_width=24  explicit_period=off  period=1  XmcBlockStatus=1  maskContainerNames=tabcontainer1  block_type=constant  block_config=sysgen:Constant_config
  Delay2 : hdlBasic/Delay  rst=off  en=off  latency=43  reg_retiming=off  XmcBlockStatus=1  maskContainerNames=group1  block_type=delay  block_config=sysgen:Delay_config
  Delay5 : hdlBasic/Delay  rst=off  en=off  latency=42  reg_retiming=off  XmcBlockStatus=1  maskContainerNames=group1  block_type=delay  block_config=sysgen:Delay_config
  Mux : hdlBasic/Mux  inputs=2  en=off  latency=0  precision=Full  arith_type=Unsigned  n_bits=16  bin_pt=14  quantization=Truncate  overflow=Wrap  XmcBlockStatus=1  maskContainerNames=tabcontainer1  block_type=mux  block_config=sysgen:Mux_config
  Mux1 : hdlBasic/Mux  inputs=2  en=off  latency=0  precision=Full  arith_type=Unsigned  n_bits=16  bin_pt=14  quantization=Truncate  overflow=Wrap  XmcBlockStatus=1  maskContainerNames=tabcontainer1  block_type=mux  block_config=sysgen:Mux_config
  Mux2 : hdlBasic/Mux  inputs=2  en=off  latency=0  precision=Full  arith_type=Unsigned  n_bits=16  bin_pt=14  quantization=Truncate  overflow=Wrap  XmcBlockStatus=1  maskContainerNames=tabcontainer1  block_type=mux  block_config=sysgen:Mux_config
  Negate11 : hdlBasic/Negate  precision=User Defined  arith_type="Signed  (2's comp)"  n_bits=16  bin_pt=13  quantization=Truncate  overflow=Wrap  en=off  latency=0  XmcBlockStatus=1  maskContainerNames=tabcontainer1  block_type=negate  block_config=sysgen:Negate_config
  Register : hdlBasic/Register  init=0  rst=on  en=off  XmcBlockStatus=1  maskContainerNames=tabcontainer1  block_type=register  block_config=sysgen:Register_config
  Scope1 : Scope
  Scope6 : Scope
  Terminator{1..7} (7 alike) : Terminator
  Vitis HLS2 : hdlBasic/Vitis HLS  anytable='C:\ELEC522\hl116\Project5\project5_final\Vitis_HLS\project5_final_hls\solution1'  fast_sim=off  display_datatype=off  rate_propagation_method=Simulink system period  model_file_path=''  latency=1  block_type=vitis_hls
      settings: infoedit=This block allows including C,C++ and SystemC source files in System Generator for DSP designs.
  theta_out : Outport
  y_out : Outport  Port=2
  x_out : Outport  Port=3
  sel_out : Outport  Port=4
  Q_out : Outport  Port=5
  Q_row4_out : Outport  Port=6
  wires:
  Mux/1 -> Mux2/3, Register/1
  Vitis HLS2/4 -> Mux/3, x_out/1
  y_in/1 -> Vitis HLS2/5
  Constant3/1 -> Mux/2
  theta_in/1 -> Delay5/1
  sel_in/1 -> Delay2/1
  Register/1 -> Vitis HLS2/4
  rst/1 -> Mux1/1, Mux2/1, Register/2
  Delay2/1 -> Mux/1, sel_out/1
  Constant6/1 -> Vitis HLS2/3
  Constant7/1 -> Vitis HLS2/7
  Constant4/1 -> Vitis HLS2/2
  Constant5/1 -> Vitis HLS2/1
  Vitis HLS2/1 -> Terminator3/1
  Vitis HLS2/2 -> Terminator1/1
  Vitis HLS2/3 -> Terminator2/1
  Vitis HLS2/5 -> Terminator4/1
  Vitis HLS2/7 -> Terminator5/1
  Vitis HLS2/8 -> Terminator6/1
  Vitis HLS2/9 -> Terminator7/1
  Mux2/1 -> Negate11/1, Scope6/1
  Mux1/1 -> Q_row4_out/1, Scope1/1
  Q_row4_in/1 -> Mux1/2
  Vitis HLS2/6 -> Mux1/3, y_out/1
  Q_in/1 -> Mux2/2
  Negate11/1 -> Q_out/1
  Delay5/1 -> theta_out/1, Vitis HLS2/6

== system QRD_System/Rotation2 ==
  y_in : Inport
  theta_in : Inport  Port=2
  rst : Inport  Port=3
  R_in : Inport  Port=4
  Constant3 : hdlBasic/Constant  const=0.0  gui_display_data_type=Fixed-point  arith_type=Signed (2's comp)  n_bits=16  bin_pt=13  preci_type=Single  exp_width=8  frac_width=24  explicit_period=off  period=1  XmcBlockStatus=1  maskContainerNames=tabcontainer1  block_type=constant  block_config=sysgen:Constant_config
  Constant4 : hdlBasic/Constant  const=1.0  gui_display_data_type=Boolean  arith_type=Boolean  n_bits=16  bin_pt=14  preci_type=Single  exp_width=8  frac_width=24  explicit_period=off  period=1  XmcBlockStatus=1  maskContainerNames=tabcontainer1  block_type=constant  block_config=sysgen:Constant_config
  Constant5 : hdlBasic/Constant  const=0  gui_display_data_type=Boolean  arith_type=Boolean  n_bits=16  bin_pt=14  preci_type=Single  exp_width=8  frac_width=24  explicit_period=off  period=1  XmcBlockStatus=1  maskContainerNames=tabcontainer1  block_type=constant  block_config=sysgen:Constant_config
  Constant6 : hdlBasic/Constant  const=0  gui_display_data_type=Boolean  arith_type=Boolean  n_bits=16  bin_pt=13  preci_type=Single  exp_width=8  frac_width=24  explicit_period=off  period=1  XmcBlockStatus=1  maskContainerNames=tabcontainer1  block_type=constant  block_config=sysgen:Constant_config
  Constant7 : hdlBasic/Constant  const=0.0  gui_display_data_type=Fixed-point  arith_type=Signed (2's comp)  n_bits=16  bin_pt=0  preci_type=Single  exp_width=8  frac_width=24  explicit_period=off  period=1  XmcBlockStatus=1  maskContainerNames=tabcontainer1  block_type=constant  block_config=sysgen:Constant_config
  Delay1 : hdlBasic/Delay  rst=off  en=off  latency=42  reg_retiming=off  XmcBlockStatus=1  maskContainerNames=group1  block_type=delay  block_config=sysgen:Delay_config
  Delay5 : hdlBasic/Delay  rst=off  en=off  latency=42  reg_retiming=off  XmcBlockStatus=1  maskContainerNames=group1  block_type=delay  block_config=sysgen:Delay_config
  Mux : hdlBasic/Mux  inputs=2  en=off  latency=0  precision=Full  arith_type=Unsigned  n_bits=16  bin_pt=14  quantization=Truncate  overflow=Wrap  XmcBlockStatus=1  maskContainerNames=tabcontainer1  block_type=mux  block_config=sysgen:Mux_config
  Mux2 : hdlBasic/Mux  inputs=2  en=off  latency=0  precision=Full  arith_type=Unsigned  n_bits=16  bin_pt=14  quantization=Truncate  overflow=Wrap  XmcBlockStatus=1  maskContainerNames=tabcontainer1  block_type=mux  block_config=sysgen:Mux_config
  Register : hdlBasic/Register  init=0  rst=on  en=off  XmcBlockStatus=1  maskContainerNames=tabcontainer1  block_type=register  block_config=sysgen:Register_config
  Scope6 : Scope
  Terminator{1..6} (6 alike) : Terminator
  Vitis HLS2 : hdlBasic/Vitis HLS  anytable='C:\ELEC522\hl116\Project5\project5_final\Vitis_HLS\project5_final_hls\solution1'  fast_sim=off  display_datatype=off  rate_propagation_method=Simulink system period  model_file_path=''  latency=1  block_type=vitis_hls
      settings: infoedit=This block allows including C,C++ and SystemC source files in System Generator for DSP designs.
  theta_out : Outport
  y_out : Outport  Port=2
  x_out : Outport  Port=3
  sel_out : Outport  Port=4
  R_out : Outport  Port=5
  rst_out : Outport  Port=6
  wires:
  Mux/1 -> Mux2/3, Register/1
  Vitis HLS2/4 -> Mux/3, x_out/1
  y_in/1 -> Vitis HLS2/5
  Constant3/1 -> Mux/2
  Vitis HLS2/5 -> Mux/1, sel_out/1
  Vitis HLS2/6 -> y_out/1
  theta_in/1 -> Delay5/1
  Register/1 -> Vitis HLS2/4
  Constant6/1 -> Vitis HLS2/3
  Constant7/1 -> Vitis HLS2/7
  Constant4/1 -> Vitis HLS2/2
  Constant5/1 -> Vitis HLS2/1
  Vitis HLS2/1 -> Terminator3/1
  Vitis HLS2/2 -> Terminator1/1
  Vitis HLS2/3 -> Terminator6/1
  Vitis HLS2/7 -> Terminator2/1
  Vitis HLS2/8 -> Terminator5/1
  Vitis HLS2/9 -> Terminator4/1
  R_in/1 -> Mux2/2
  rst/1 -> Delay1/1, Mux2/1, Register/2
  Mux2/1 -> R_out/1, Scope6/1
  Delay5/1 -> theta_out/1, Vitis HLS2/6
  Delay1/1 -> rst_out/1

== system QRD_System/Rotation3 ==
  y_in : Inport
  theta_in : Inport  Port=2
  sel_in : Inport  Port=3
  rst : Inport  Port=4
  R_in : Inport  Port=5
  Constant3 : hdlBasic/Constant  const=0.0  gui_display_data_type=Fixed-point  arith_type=Signed (2's comp)  n_bits=16  bin_pt=13  preci_type=Single  exp_width=8  frac_width=24  explicit_period=off  period=1  XmcBlockStatus=1  maskContainerNames=tabcontainer1  block_type=constant  block_config=sysgen:Constant_config
  Constant4 : hdlBasic/Constant  const=1.0  gui_display_data_type=Boolean  arith_type=Boolean  n_bits=16  bin_pt=14  preci_type=Single  exp_width=8  frac_width=24  explicit_period=off  period=1  XmcBlockStatus=1  maskContainerNames=tabcontainer1  block_type=constant  block_config=sysgen:Constant_config
  Constant5 : hdlBasic/Constant  const=0  gui_display_data_type=Boolean  arith_type=Boolean  n_bits=16  bin_pt=14  preci_type=Single  exp_width=8  frac_width=24  explicit_period=off  period=1  XmcBlockStatus=1  maskContainerNames=tabcontainer1  block_type=constant  block_config=sysgen:Constant_config
  Constant6 : hdlBasic/Constant  const=0  gui_display_data_type=Boolean  arith_type=Boolean  n_bits=16  bin_pt=13  preci_type=Single  exp_width=8  frac_width=24  explicit_period=off  period=1  XmcBlockStatus=1  maskContainerNames=tabcontainer1  block_type=constant  block_config=sysgen:Constant_config
  Constant7 : hdlBasic/Constant  const=0.0  gui_display_data_type=Fixed-point  arith_type=Signed (2's comp)  n_bits=16  bin_pt=0  preci_type=Single  exp_width=8  frac_width=24  explicit_period=off  period=1  XmcBlockStatus=1  maskContainerNames=tabcontainer1  block_type=constant  block_config=sysgen:Constant_config
  Delay1 : hdlBasic/Delay  rst=off  en=off  latency=42  reg_retiming=off  XmcBlockStatus=1  maskContainerNames=group1  block_type=delay  block_config=sysgen:Delay_config
  Delay2 : hdlBasic/Delay  rst=off  en=off  latency=43  reg_retiming=off  XmcBlockStatus=1  maskContainerNames=group1  block_type=delay  block_config=sysgen:Delay_config
  Delay5 : hdlBasic/Delay  rst=off  en=off  latency=0  reg_retiming=off  XmcBlockStatus=1  maskContainerNames=group1  block_type=delay  block_config=sysgen:Delay_config
  Mux : hdlBasic/Mux  inputs=2  en=off  latency=0  precision=Full  arith_type=Unsigned  n_bits=16  bin_pt=14  quantization=Truncate  overflow=Wrap  XmcBlockStatus=1  maskContainerNames=tabcontainer1  block_type=mux  block_config=sysgen:Mux_config
  Mux2 : hdlBasic/Mux  inputs=2  en=off  latency=0  precision=Full  arith_type=Unsigned  n_bits=16  bin_pt=14  quantization=Truncate  overflow=Wrap  XmcBlockStatus=1  maskContainerNames=tabcontainer1  block_type=mux  block_config=sysgen:Mux_config
  Register : hdlBasic/Register  init=0  rst=on  en=off  XmcBlockStatus=1  maskContainerNames=tabcontainer1  block_type=register  block_config=sysgen:Register_config
  Scope6 : Scope
  Terminator{1..7} (7 alike) : Terminator
  Vitis HLS2 : hdlBasic/Vitis HLS  anytable='C:\ELEC522\hl116\Project5\project5_final\Vitis_HLS\project5_final_hls\solution1'  fast_sim=off  display_datatype=off  rate_propagation_method=Simulink system period  model_file_path=''  latency=1  block_type=vitis_hls
      settings: infoedit=This block allows including C,C++ and SystemC source files in System Generator for DSP designs.
  theta_out : Outport
  y_out : Outport  Port=2
  x_out : Outport  Port=3
  R_out : Outport  Port=4
  rst_out : Outport  Port=5
  wires:
  Vitis HLS2/4 -> Mux/3, x_out/1
  y_in/1 -> Vitis HLS2/5
  Constant3/1 -> Mux/2
  Vitis HLS2/6 -> y_out/1
  sel_in/1 -> Delay2/1
  rst/1 -> Delay1/1, Mux2/1, Register/2
  Mux/1 -> Mux2/3, Register/1
  Register/1 -> Vitis HLS2/4
  Constant6/1 -> Vitis HLS2/3
  Constant7/1 -> Vitis HLS2/7
  Constant4/1 -> Vitis HLS2/2
  Constant5/1 -> Vitis HLS2/1
  theta_in/1 -> Delay5/1
  Vitis HLS2/5 -> Terminator4/1
  Vitis HLS2/7 -> Terminator5/1
  Vitis HLS2/8 -> Terminator6/1
  Vitis HLS2/9 -> Terminator7/1
  Vitis HLS2/2 -> Terminator1/1
  Vitis HLS2/1 -> Terminator3/1
  Vitis HLS2/3 -> Terminator2/1
  Delay2/1 -> Mux/1
  Mux2/1 -> R_out/1, Scope6/1
  R_in/1 -> Mux2/2
  Delay5/1 -> theta_out/1, Vitis HLS2/6
  Delay1/1 -> rst_out/1
